simulink model "CruiseControl3"  (Simulink 5.0)
settings: Solver=ode45  SolverMode=SingleTasking  StartTime=0.0  StopTime=150.0  RelTol=1e-3
PreLoadFcn:
  | load cruise_data;
undefined symbols (not defined in the file): emap, Iei, Ki, Kp, SpeedInc, SpeedMax, SpeedMin, Ts
settings Model: Creator=Esterel Technologies  LastModifiedBy=scaife  ExtModeTrigMode=oneshot  ExtModeArmWhenConnect=off  ExtModeAutoUpdateStatusClock=off  SaveTime=off  SaveOutput=off  LimitDataPoints=off  MaxDataPoints=10000  BooleanDataType=off

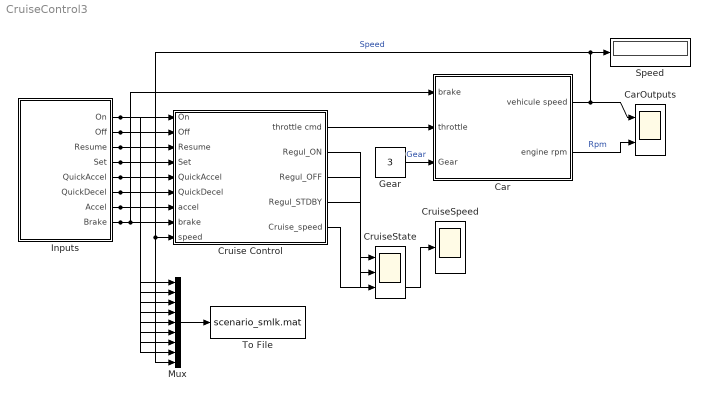
== system CruiseControl3 ==
  Car : Subsystem
      mask Display: plot([cos(pi*[0:5:360]/180) + 6], [sin(pi*[0:5:360]/180) + 1.5],[cos(pi*[0:5:360]/180) + 1], [sin(pi*[0:5:360]/180) + 4], [10 7.5 6.75], [3.5 1 1.5], [10 9.75 7.5 6.25 3 1.5 4 5 7.5], [3.5 4.75 5.5 7 8 7 6 4 5.5], [6.5 4], [7 6], [5.25 2], [2 4], [7.5 1 0], [2.5 6 6.5], [7.5 7.25 9.75], [1 2.25 4.75], [2.75 2 0 0 0.25], [7.5 8 6.5 5.25 5], [1.5 0.5], [6.75 6.25])
  CarOutputs : Scope  NumInputPorts=2
      settings: TickLabels=on  YMin=-25~500  YMax=150~6000  DataFormat=Array
  Cruise Control : Subsystem
  CruiseSpeed : Scope
      settings: TickLabels=on  YMin=-25  YMax=150  DataFormat=Array
  CruiseState : Scope  NumInputPorts=3
      settings: TickLabels=on  YMin=-1~-1~-1  YMax=2~2~2  DataFormat=Array
  Gear : Constant  Value=3
  Inputs : Subsystem
  Mux : Mux  Inputs=9
  Speed : Display
  To File : ToFile  Filename=scenario_smlk.mat  SampleTime=0.3333
  wires:
  Cruise Control/1(throttle cmd) -> Car/2(throttle)
  Car/1(vehicule speed) -> CarOutputs/1, Speed/1, Cruise Control/9(speed), Mux/9  "Speed"
  Car/2(engine rpm) -> CarOutputs/2  "Rpm"
  Cruise Control/2(Regul_ON) -> CruiseState/1
  Cruise Control/3(Regul_OFF) -> CruiseState/2
  Cruise Control/4(Regul_STDBY) -> CruiseState/3
  Cruise Control/5(Cruise_speed) -> CruiseSpeed/1
  Mux/1 -> To File/1
  Inputs/1(On) -> Mux/1, Cruise Control/1(On)
  Inputs/2(Off) -> Mux/2, Cruise Control/2(Off)
  Inputs/3(Resume) -> Mux/3, Cruise Control/3(Resume)
  Inputs/4(Set) -> Mux/4, Cruise Control/4(Set)
  Inputs/5(QuickAccel) -> Mux/5, Cruise Control/5(QuickAccel)
  Inputs/6(QuickDecel) -> Mux/6, Cruise Control/6(QuickDecel)
  Inputs/7(Accel) -> Mux/7, Cruise Control/7(accel)
  Inputs/8(Brake) -> Mux/8, Cruise Control/8(brake), Car/1(brake)
  Gear/1 -> Car/3(Gear)  "Gear"

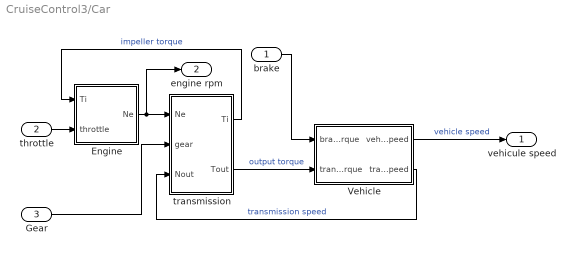
== system CruiseControl3/Car ==
  brake : Inport
  throttle : Inport  Port=2
  Gear : Inport  Port=3
  Engine : Subsystem
  Vehicle : Subsystem  mask(vehicle model){Rfd=3.23, rload0=40, rload2=0.02, Rw=1, Iv=12.0941, N20=0}
      mask prompts: Rfd "final drive ratio"; rload0 "drag friction at wheels"; rload2 "aerodynamic drag"; Rw "wheel radius"; Iv "vehicle inertia"; N20 "initial transmission output speed"
      mask help: vehicle dynamics: torque input from trans., outputs are input speed (transmission output) and vehicle speed
      mask Display: plot([cos(pi*[0:5:360]/180) + 6], [sin(pi*[0:5:360]/180) + 1.5],[cos(pi*[0:5:360]/180) + 1], [sin(pi*[0:5:360]/180) + 4], [10 7.5 6.75], [3.5 1 1.5], [10 9.75 7.5 6.25 3 1.5 4 5 7.5], [3.5 4.75 5.5 7 8 7 6 4 5.5], [6.5 4], [7 6], [5.25 2], [2 4], [7.5 1 0], [2.5 6 6.5], [7.5 7.25 9.75], [1 2.25 4.75], [2.75 2 0 0 0.25], [7.5 8 6.5 5.25 5], [1.5 0.5], [6.75 6.25])
  transmission : Subsystem
  vehicule speed : Outport
  engine rpm : Outport  Port=2
  wires:
  transmission/1(Ti) -> Engine/1(Ti)  "impeller torque"
  transmission/2(Tout) -> Vehicle/2(transmission output torque)  "output torque"
  Vehicle/2(transmission output speed) -> transmission/3(Nout)  "transmission speed"
  throttle/1 -> Engine/2(throttle)
  Vehicle/1(vehicle speed) -> vehicule speed/1  "vehicle speed"
  brake/1 -> Vehicle/1(brake torque)
  Gear/1 -> transmission/2(gear)
  Engine/1(Ne) -> transmission/1(Ne), engine rpm/1

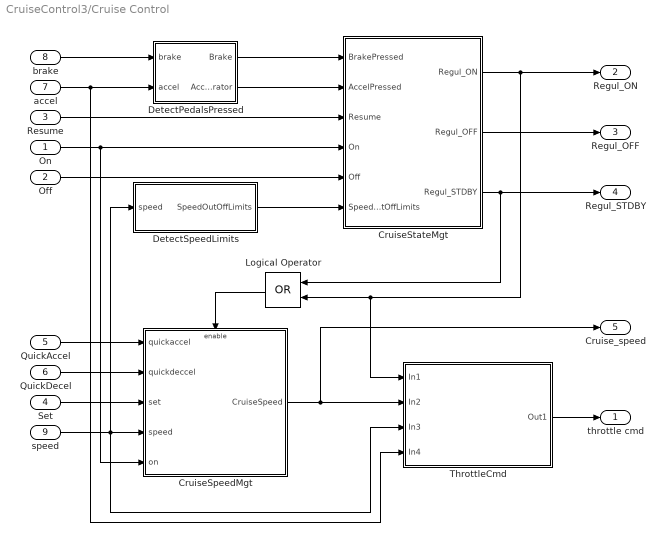
== system CruiseControl3/Cruise Control ==
  On : Inport  SampleTime=Ts
  Off : Inport  Port=2  SampleTime=Ts
  Resume : Inport  Port=3  SampleTime=Ts
  Set : Inport  Port=4  SampleTime=Ts
  QuickAccel : Inport  Port=5  SampleTime=Ts
  QuickDecel : Inport  Port=6  SampleTime=Ts
  accel : Inport  Port=7  SampleTime=Ts
  brake : Inport  Port=8  SampleTime=Ts
  speed : Inport  Port=9  SampleTime=Ts
  CruiseSpeedMgt : Subsystem  TreatAsAtomicUnit=on
  CruiseStateMgt : Stateflow chart
  DetectPedalsPressed : Subsystem
  DetectSpeedLimits : Subsystem
  Logical Operator : Logic  Orientation=left  Operator=OR
  ThrottleCmd : Subsystem
  throttle cmd : Outport
  Regul_ON : Outport  Port=2
  Regul_OFF : Outport  Port=3
  Regul_STDBY : Outport  Port=4
  Cruise_speed : Outport  Port=5
  wires:
  Resume/1 -> CruiseStateMgt/3(Resume)
  Off/1 -> CruiseStateMgt/5(Off)
  CruiseStateMgt/1(Regul_ON) -> Regul_ON/1, Logical Operator/2, ThrottleCmd/1(In1)
  QuickAccel/1 -> CruiseSpeedMgt/1(quickaccel)
  Logical Operator/1 -> CruiseSpeedMgt/Enable
  QuickDecel/1 -> CruiseSpeedMgt/2(quickdeccel)
  Set/1 -> CruiseSpeedMgt/3(set)
  DetectPedalsPressed/1(Brake) -> CruiseStateMgt/1(BrakePressed)
  DetectPedalsPressed/2(Accelerator) -> CruiseStateMgt/2(AccelPressed)
  accel/1 -> DetectPedalsPressed/2(accel), ThrottleCmd/4(In4)
  brake/1 -> DetectPedalsPressed/1(brake)
  ThrottleCmd/1(Out1) -> throttle cmd/1
  CruiseStateMgt/2(Regul_OFF) -> Regul_OFF/1
  CruiseStateMgt/3(Regul_STDBY) -> Logical Operator/1, Regul_STDBY/1
  On/1 -> CruiseSpeedMgt/5(on), CruiseStateMgt/4(On)
  CruiseSpeedMgt/1(CruiseSpeed) -> Cruise_speed/1, ThrottleCmd/2(In2)
  speed/1 -> CruiseSpeedMgt/4(speed), DetectSpeedLimits/1(speed), ThrottleCmd/3(In3)
  DetectSpeedLimits/1(SpeedOutOffLimits) -> CruiseStateMgt/6(SpeedOutOffLimits)

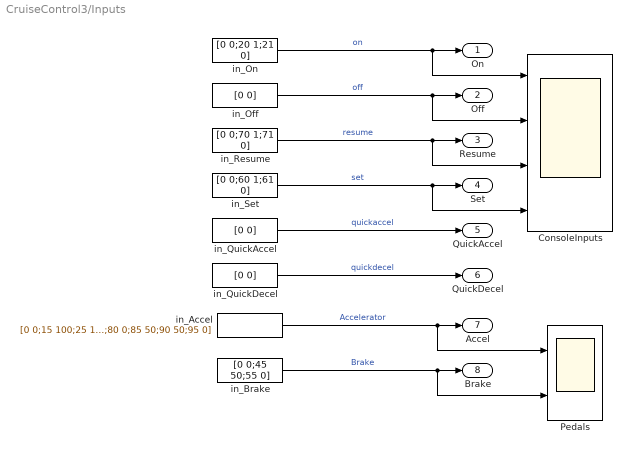
== system CruiseControl3/Inputs ==
  ConsoleInputs : Scope  NumInputPorts=4
      settings: TickLabels=on  YMin=-5~-5~-5~-5  YMax=5~5~5~5
  Pedals : Scope  NumInputPorts=2
      settings: TickLabels=on  YMin=-900~-1  YMax=100~1  SaveName=ScopeData2
  in_Accel : FromWorkspace  VariableName=[0 0;15 100;25 100;26 0;80 0;85 50;90 50;95 0]  SampleTime=0.2  OutputAfterFinalValue=Holding final value
  in_Brake : FromWorkspace  VariableName=[0 0;45 50;55 0]  SampleTime=0.2  Interpolate=off  OutputAfterFinalValue=Holding final value
  in_Off : FromWorkspace  VariableName=[0 0]  SampleTime=0.2  Interpolate=off  OutputAfterFinalValue=Holding final value
  in_On : FromWorkspace  VariableName=[0 0;20 1;21 0]  SampleTime=0.2  Interpolate=off  OutputAfterFinalValue=Holding final value
  in_QuickAccel : FromWorkspace  VariableName=[0 0]  SampleTime=0.2  Interpolate=off  OutputAfterFinalValue=Holding final value
  in_QuickDecel : FromWorkspace  VariableName=[0 0]  SampleTime=0.2  Interpolate=off  OutputAfterFinalValue=Holding final value
  in_Resume : FromWorkspace  VariableName=[0 0;70 1;71 0]  SampleTime=0.2  Interpolate=off  OutputAfterFinalValue=Holding final value
  in_Set : FromWorkspace  VariableName=[0 0;60 1;61 0]  SampleTime=0.2  Interpolate=off  OutputAfterFinalValue=Holding final value
  On : Outport
  Off : Outport  Port=2
  Resume : Outport  Port=3
  Set : Outport  Port=4
  QuickAccel : Outport  Port=5
  QuickDecel : Outport  Port=6
  Accel : Outport  Port=7
  Brake : Outport  Port=8
  wires:
  in_Resume/1 -> Resume/1, ConsoleInputs/3  "resume"
  in_On/1 -> On/1, ConsoleInputs/1  "on"
  in_Off/1 -> Off/1, ConsoleInputs/2  "off"
  in_QuickAccel/1 -> QuickAccel/1  "quickaccel"
  in_QuickDecel/1 -> QuickDecel/1  "quickdecel"
  in_Set/1 -> Set/1, ConsoleInputs/4  "set"
  in_Brake/1 -> Brake/1, Pedals/2  "Brake"
  in_Accel/1 -> Accel/1, Pedals/1  "Accelerator"

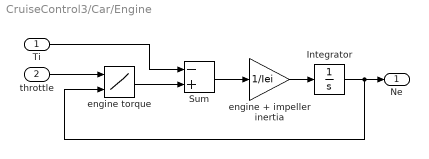
== system CruiseControl3/Car/Engine ==
  Ti : Inport
  throttle : Inport  Port=2
  Integrator : Integrator  InitialCondition=1000  LimitOutput=on  UpperSaturationLimit=6000  LowerSaturationLimit=600
  Sum : Sum  Inputs=-+  SaturateOnIntegerOverflow=on  InputSameDT=on
  engine torque : Lookup2D  RowIndex=thvec  ColumnIndex=nevec  OutputValues=emap  SaturateOnIntegerOverflow=on  InputSameDT=on
  engine + impeller inertia : Gain  Gain=1/Iei  SaturateOnIntegerOverflow=on
  Ne : Outport  InitialOutput=0
  wires:
  engine torque/1 -> Sum/2
  engine + impeller inertia/1 -> Integrator/1
  Sum/1 -> engine + impeller inertia/1
  Integrator/1 -> Ne/1, engine torque/2
  throttle/1 -> engine torque/1
  Ti/1 -> Sum/1

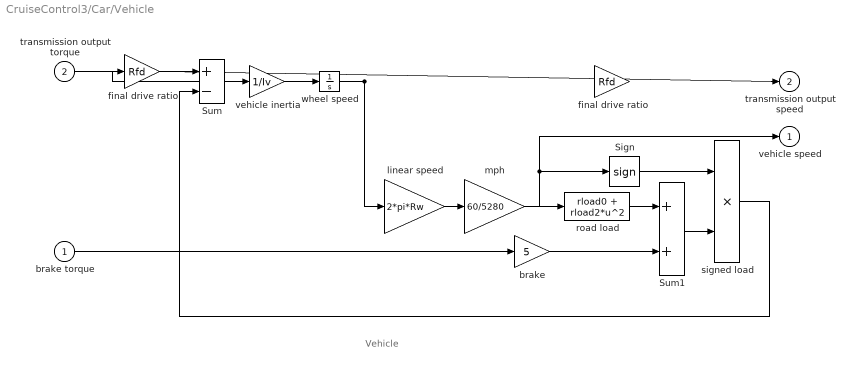
== system CruiseControl3/Car/Vehicle ==
  note: Vehicle
  brake torque : Inport
  transmission output torque : Inport  Port=2
  Sign : Signum
  Sum : Sum  Inputs=+-  SaturateOnIntegerOverflow=on  InputSameDT=on
  Sum1 : Sum  SaturateOnIntegerOverflow=on  InputSameDT=on
  brake : Gain  Gain=5  SaturateOnIntegerOverflow=on
  final drive ratio : Gain  Gain=Rfd  SaturateOnIntegerOverflow=on
  final drive ratio : Gain  Gain=Rfd  SaturateOnIntegerOverflow=on
  linear speed : Gain  Gain=2*pi*Rw  SaturateOnIntegerOverflow=on
  mph : Gain  Gain=60/5280  SaturateOnIntegerOverflow=on
  road load : Fcn  Expr=rload0 + rload2*u^2
  signed load : Product  SaturateOnIntegerOverflow=on  InputSameDT=on
  vehicle inertia : Gain  Gain=1/Iv  SaturateOnIntegerOverflow=on
  wheel speed : Integrator  InitialCondition=N20/Rfd
  vehicle speed : Outport  InitialOutput=0
  transmission output speed : Outport  Port=2  InitialOutput=0
  wires:
  final drive ratio/1 -> Sum/1
  wheel speed/1 -> final drive ratio/1, linear speed/1
  linear speed/1 -> mph/1
  mph/1 -> road load/1, Sign/1, vehicle speed/1
  Sum/1 -> vehicle inertia/1
  vehicle inertia/1 -> wheel speed/1
  transmission output torque/1 -> final drive ratio/1
  signed load/1 -> Sum/2
  Sign/1 -> signed load/1
  road load/1 -> Sum1/1
  Sum1/1 -> signed load/2
  final drive ratio/1 -> transmission output speed/1
  brake torque/1 -> brake/1
  brake/1 -> Sum1/2

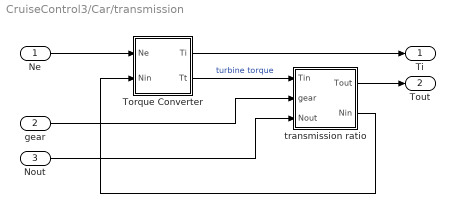
== system CruiseControl3/Car/transmission ==
  Ne : Inport
  gear : Inport  Port=2
  Nout : Inport  Port=3
  Torque Converter : Subsystem  mask(torque converter){speedratio=[0    0.1000    0.2000    0.3000    0.4000    0.5000    0.6000 0.7000    0.8000    0.8100    0.8200    0.8300    0.8400    0.8500 0.8600    0.8700    0.8800    0.8900    0.9000    0.9200    0.9400], Kfactor=[137.4652  137.0650  135.8644  135.6644  137.5653  140.3666  145.2689 152.8725  162.9773  164.2779  166.1788  167.9797  170.0807  172.7820 175.3832  179.5852  183.5871  189.8901  197.6938  215.9024  244.5160], Torkratio=[2.2320    2.0750    1.9750    1.8460    1.7200    1.5640    1.4090 1.2540    1.0960    1.0800    1.0610    1.0430    1.0280    1.0120 1.0020    1.0020    1.0010    0.9980    0.9990    1.0010    1.0020]}
      mask prompts: speedratio "speed ratio"; Kfactor "K factor"; Torkratio "torque ratio"
      mask help: torque converter
      mask Help: Torque converter input and output torques are computed as a function of the input and output speeds
      mask Display: plot([cos([90:10:450]*pi/180),.63*cos([90:10:450]*pi/180),.63*cos([90:10:240]*pi/180),cos([240:10:300]*pi/180),.63*cos([300]*pi/180)],[sin([90:10:450]*pi/180),.63*sin([90:10:450]*pi/180)+.1,.63*sin([90:10:240]*pi/180)+.1,sin([240:10:300]*pi/180),.63*sin([300]*pi/180)+.1])
  transmission ratio : Subsystem
  Ti : Outport  InitialOutput=0
  Tout : Outport  Port=2  InitialOutput=0
  wires:
  Torque Converter/2(Tt) -> transmission ratio/1(Tin)  "turbine torque"
  transmission ratio/2(Nin) -> Torque Converter/2(Nin)
  Ne/1 -> Torque Converter/1(Ne)
  gear/1 -> transmission ratio/2(gear)
  Nout/1 -> transmission ratio/3(Nout)
  Torque Converter/1(Ti) -> Ti/1
  transmission ratio/1(Tout) -> Tout/1

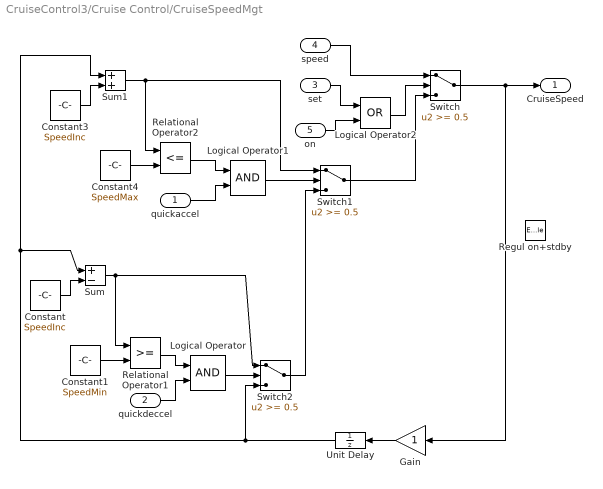
== system CruiseControl3/Cruise Control/CruiseSpeedMgt ==
  quickaccel : Inport
  quickdeccel : Inport  Port=2
  set : Inport  Port=3
  speed : Inport  Port=4
  on : Inport  Port=5
  Regul on+stdby : EnablePort
  Constant : Constant  Value=SpeedInc
  Constant1 : Constant  Value=SpeedMin
  Constant3 : Constant  Value=SpeedInc
  Constant4 : Constant  Value=SpeedMax
  Gain : Gain  Orientation=left  SaturateOnIntegerOverflow=on
  Logical Operator : Logic
  Logical Operator1 : Logic
  Logical Operator2 : Logic  Operator=OR
  Relational Operator1 : RelationalOperator  InputSameDT=on
  Relational Operator2 : RelationalOperator  Operator=<=  InputSameDT=on
  Sum : Sum  Inputs=+-  SaturateOnIntegerOverflow=on  InputSameDT=on
  Sum1 : Sum  SaturateOnIntegerOverflow=on  InputSameDT=on
  Switch : Switch  Threshold=0.5  SaturateOnIntegerOverflow=on  InputSameDT=on
  Switch1 : Switch  Threshold=0.5  SaturateOnIntegerOverflow=on  InputSameDT=on
  Switch2 : Switch  Threshold=0.5  SaturateOnIntegerOverflow=on  InputSameDT=on
  Unit Delay : UnitDelay  Orientation=left  SampleTime=0.1
  CruiseSpeed : Outport
  wires:
  speed/1 -> Switch/1
  Relational Operator1/1 -> Logical Operator/1
  quickdeccel/1 -> Logical Operator/2
  Constant1/1 -> Relational Operator1/2
  Sum/1 -> Relational Operator1/1, Switch2/1
  Unit Delay/1 -> Switch2/3, Sum/1, Sum1/1
  Relational Operator2/1 -> Logical Operator1/1
  Constant4/1 -> Relational Operator2/2
  Sum1/1 -> Relational Operator2/1, Switch1/1
  quickaccel/1 -> Logical Operator1/2
  Switch1/1 -> Switch/3
  Switch2/1 -> Switch1/3
  Logical Operator/1 -> Switch2/2
  Logical Operator1/1 -> Switch1/2
  set/1 -> Logical Operator2/1
  Gain/1 -> Unit Delay/1
  Switch/1 -> CruiseSpeed/1, Gain/1
  on/1 -> Logical Operator2/2
  Logical Operator2/1 -> Switch/2
  Constant3/1 -> Sum1/2
  Constant/1 -> Sum/2

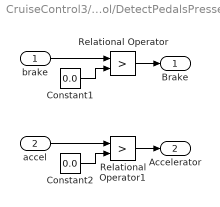
== system CruiseControl3/Cruise Control/DetectPedalsPressed ==
  brake : Inport
  accel : Inport  Port=2
  Constant1 : Constant  Value=0.0
  Constant2 : Constant  Value=0.0
  Relational Operator : RelationalOperator  Operator=>  InputSameDT=on
  Relational Operator1 : RelationalOperator  Operator=>  InputSameDT=on
  Brake : Outport
  Accelerator : Outport  Port=2
  wires:
  Constant1/1 -> Relational Operator/2
  brake/1 -> Relational Operator/1
  Relational Operator/1 -> Brake/1
  Constant2/1 -> Relational Operator1/2
  accel/1 -> Relational Operator1/1
  Relational Operator1/1 -> Accelerator/1

== system CruiseControl3/Cruise Control/DetectSpeedLimits ==
  speed : Inport
  Constant : Constant  Value=SpeedMin
  Constant1 : Constant  Value=SpeedMax
  Logical Operator : Logic  Operator=OR
  Relational Operator : RelationalOperator  Operator=<  InputSameDT=on
  Relational Operator1 : RelationalOperator  Operator=>  InputSameDT=on
  SpeedOutOffLimits : Outport
  wires:
  Constant1/1 -> Relational Operator1/2
  Constant/1 -> Relational Operator/2
  speed/1 -> Relational Operator1/1, Relational Operator/1
  Logical Operator/1 -> SpeedOutOffLimits/1
  Relational Operator/1 -> Logical Operator/1
  Relational Operator1/1 -> Logical Operator/2

== system CruiseControl3/Cruise Control/ThrottleCmd ==
  In1 : Inport
  In2 : Inport  Port=2
  In3 : Inport  Port=3
  In4 : Inport  Port=4
  Regulator : Subsystem  TreatAsAtomicUnit=on
  Switch : Switch  Threshold=0.5  SaturateOnIntegerOverflow=on  InputSameDT=on
  Out1 : Outport
  wires:
  Regulator/1(Cmd) -> Switch/1
  In2/1 -> Regulator/1(Cruise Speed)
  In3/1 -> Regulator/2(Speed)
  In4/1 -> Switch/3
  Switch/1 -> Out1/1
  In1/1 -> Regulator/Enable, Switch/2

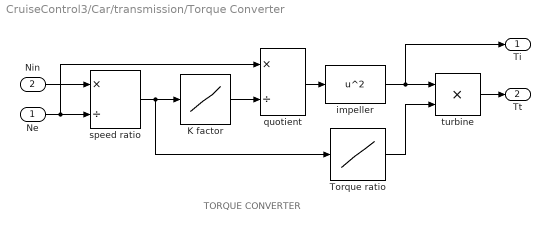
== system CruiseControl3/Car/transmission/Torque Converter ==
  note: TORQUE CONVERTER
  Ne : Inport
  Nin : Inport  Port=2
  K factor : Lookup  InputValues=speedratio  OutputValues=Kfactor  SaturateOnIntegerOverflow=on
  Torque ratio : Lookup  InputValues=speedratio  OutputValues=Torkratio  SaturateOnIntegerOverflow=on
  impeller : Fcn  Expr=u^2
  quotient : Product  Inputs=*/  SaturateOnIntegerOverflow=on  InputSameDT=on
  speed ratio : Product  Inputs=*/  SaturateOnIntegerOverflow=on  InputSameDT=on
  turbine : Product  SaturateOnIntegerOverflow=on  InputSameDT=on
  Ti : Outport  InitialOutput=0
  Tt : Outport  Port=2  InitialOutput=0
  wires:
  Nin/1 -> speed ratio/1
  Ne/1 -> quotient/1, speed ratio/2
  turbine/1 -> Tt/1
  impeller/1 -> Ti/1, turbine/1
  speed ratio/1 -> K factor/1, Torque ratio/1
  K factor/1 -> quotient/2
  quotient/1 -> impeller/1
  Torque ratio/1 -> turbine/2

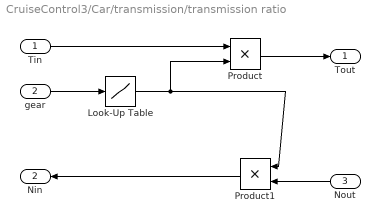
== system CruiseControl3/Car/transmission/transmission ratio ==
  Tin : Inport
  gear : Inport  Port=2
  Nout : Inport  Orientation=left  Port=3
  Look-Up Table : Lookup  InputValues=[1 2 3 4]  OutputValues=[2.393 1.45 1.0 0.677]  SaturateOnIntegerOverflow=on
  Product : Product  SaturateOnIntegerOverflow=on  InputSameDT=on
  Product1 : Product  Orientation=left  SaturateOnIntegerOverflow=on  InputSameDT=on
  Tout : Outport  InitialOutput=0
  Nin : Outport  Orientation=left  Port=2  InitialOutput=0
  wires:
  gear/1 -> Look-Up Table/1
  Tin/1 -> Product/1
  Product/1 -> Tout/1
  Product1/1 -> Nin/1
  Nout/1 -> Product1/2
  Look-Up Table/1 -> Product/2, Product1/1

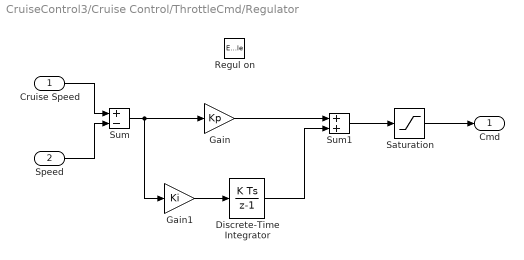
== system CruiseControl3/Cruise Control/ThrottleCmd/Regulator ==
  Cruise Speed : Inport
  Speed : Inport  Port=2
  Regul on : EnablePort
  Discrete-Time Integrator : DiscreteIntegrator  LimitOutput=on  UpperSaturationLimit=200  LowerSaturationLimit=-10  SampleTime=0.1
  Gain : Gain  Gain=Kp  SaturateOnIntegerOverflow=on
  Gain1 : Gain  Gain=Ki  SaturateOnIntegerOverflow=on
  Saturation : Saturate  UpperLimit=50  LowerLimit=0
  Sum : Sum  Inputs=+-  SaturateOnIntegerOverflow=on  InputSameDT=on
  Sum1 : Sum  SaturateOnIntegerOverflow=on  InputSameDT=on
  Cmd : Outport
  wires:
  Gain/1 -> Sum1/1
  Gain1/1 -> Discrete-Time Integrator/1
  Sum/1 -> Gain/1, Gain1/1
  Sum1/1 -> Saturation/1
  Saturation/1 -> Cmd/1
  Discrete-Time Integrator/1 -> Sum1/2
  Cruise Speed/1 -> Sum/1
  Speed/1 -> Sum/2

== stateflow chart Cruise Control/CruiseStateMgt ==
  settings: updateMethod=DISCRETE  sampleTime=0.2
  state Disabled
    entry:
    Regul_OFF = 1;
    Regul_ON = 0;
    Regul_STDBY = 0
  state Enabled
    state Interrupted
      entry:
      Regul_OFF = 1;
      Regul_ON = 0;
      Regul_STDBY = 1
    state Regulation
      state On
        entry:
        Regul_OFF = 0;
        Regul_ON = 1;
        Regul_STDBY = 0
      state StandBy
        entry:
        Regul_OFF = 0;
        Regul_ON = 0;
        Regul_STDBY = 1
      (junction 9) -> StandBy : [AccelPressed  | SpeedOutOffLimits ]
      On -> StandBy : [AccelPressed  | SpeedOutOffLimits ]
      StandBy -> On : [~AccelPressed & ~SpeedOutOffLimits]
      (junction 9) -> On
      (default) -> (junction 9)
    Regulation -> Interrupted : [BrakePressed]
    Interrupted -> Regulation : [Resume & ~BrakePressed]
    (default) -> (junction 10)
    (junction 10) -> Interrupted : [BrakePressed]
    (junction 10) -> Regulation
  (default) -> (junction 11)
  Disabled -> Enabled : [On]
  Enabled -> Disabled : [Off]
  (junction 11) -> Disabled
  (junction 11) -> Enabled : [On]
  data: BrakePressed input boolean; AccelPressed input boolean; Resume input boolean; On input boolean; Off input boolean; SpeedOutOffLimits input boolean; Regul_ON output boolean; Regul_OFF output boolean; Regul_STDBY output boolean
